simulink model "CurrentWithoutSim"  (R2022b)
settings: Solver=VariableStepAuto  StartTime=0.0  StopTime=20  RelTol=1e-3
PreLoadFcn:
  | openManipulatorParameters;
PostLoadFcn:
  | % Insert Communication Stuff Here
StartFcn:
  | myDxl.doEnableTorque(11);
  | myDxl.doEnableTorque(12);
  | myDxl.doEnableTorque(13);
  | myDxl.doEnableTorque(14);
  | myDxl.doEnableTorque(15);
StopFcn:
  | myDxl.doDisableTorque(11);
  | myDxl.doDisableTorque(12);
  | myDxl.doDisableTorque(13);
  | myDxl.doDisableTorque(14);
  | myDxl.doDisableTorque(15);
undefined symbols (not defined in the file): group_num_read, group_num_write, TsCtrl
libraries: slDxl_lib x12, dxlSimLibrary x2, OpenManipulatorLib x1
CloseFcn:
  | myDxl.delete()
settings Model: Creator=scastro  LastModifiedBy=Boog
settings SolverCC: AlgebraicLoopSolver=TrustRegion  DecoupledContinuousIntegration=on  MinimalZcImpactIntegration=on
settings DataIOCC: ReturnWorkspaceOutputs=off
settings DebuggingCC: ParameterOverflowMsg=none  UnconnectedInputMsg=warning  UnconnectedOutputMsg=warning  UnconnectedLineMsg=warning  SFMachineParentedDataDiag=warning  ArithmeticOperatorsInVariantConditions=warning
settings ModelReferenceCC: EnableRefExpFcnMdlSchedulingChecks=on
settings SFSimCC: SimUseLocalCustomCode=off  CustomCodeUndefinedFunction=UseInterfaceOnly
settings RTWCC: RTWUseLocalCustomCode=off
settings ExplorerConfigSet: InternalSimMechanicsExplorerSettings="<ExplorerConfiguration><canonicalview>default</canonicalview><AnimationSetting><BasePlaybackSpeed>1.0</BasePlaybackSpeed><PlaybackSpeedFactor>1.0</PlaybackSpeedFactor></AnimationSetting><TilePanel><TileInfo><Tiles Columns=\"1\" Count=\"1\" Rows=\"1\"><Column Weight=\"1\"/><Row Weight=\"1\"/><Tile Height=\"1\" Width=\"1\" X=\"0\" Y=\"0\"/></Tiles></TileInfo><SceneInfo><SceneViewer><BGColor><R>0.60000002384185791</R><G>0.60000002384185791</G><B>0.60000002384185791</B></BGColor><Camera><DoPerspective>off</DoPerspective><Position><X>0.428752942017998073</X><Y>-0.712150369953937545</Y><Z>0.628314823463847372</Z></Position><Center><X>0.0455703138120887447</X><Y>0.0802507835591396851</Y><Z>0.153687090021758288</Z></Center><Up><X>-0.128866037345358619</X><Y>0.462960972240881619</Y><Z>0.876961049648547597</Z></Up><ViewLimDist>1</ViewLimDist><YLim>0.579070269035580121</YLim><XLim>0.64437894599448009</XLim></Camera></SceneViewer></SceneInfo></TilePanel><MechEditorPanel><Cameras/><GfxPanelCameraMap/><VideoCreator><PlaybackSpeedRatio>1.0</PlaybackSpeedRatio><FrameRate>30</FrameRate><VideoFormat>Motion JPEG AVI</VideoFormat><FrameSize>auto</FrameSize></VideoCreator></MechEditorPanel></ExplorerConfiguration>"

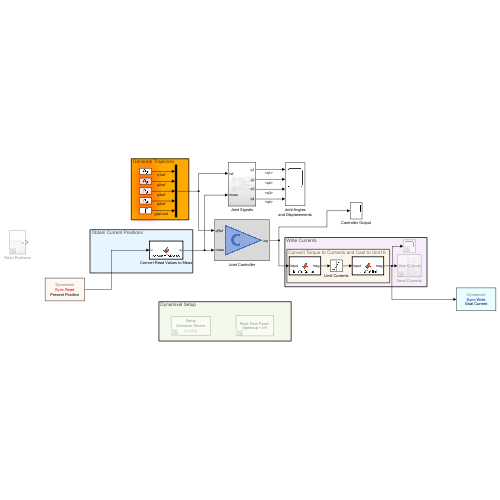
[thumbnail: Simulink's stored preview of the top-level diagram]
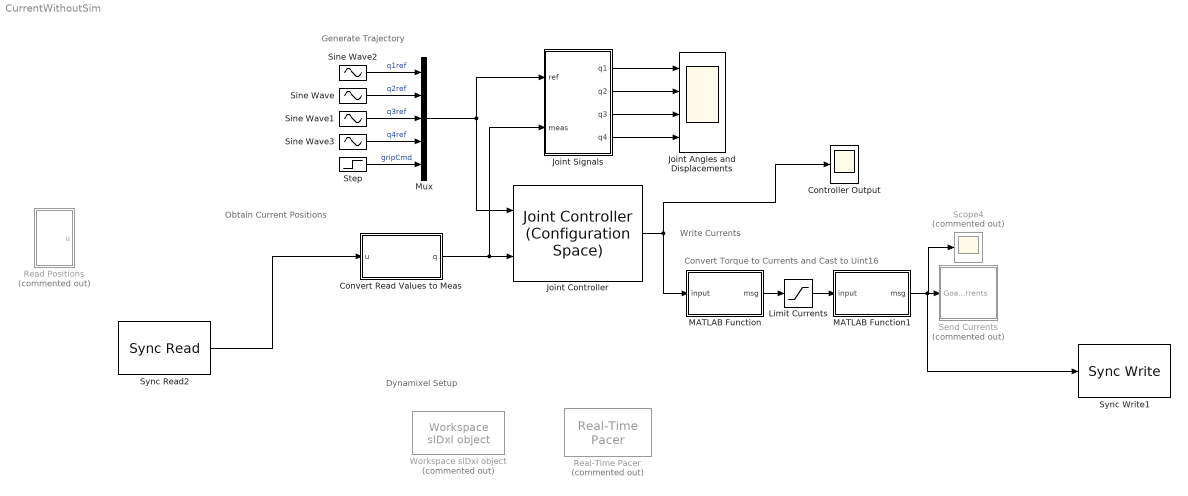
== system CurrentWithoutSim ==
  note: Dynamixel Setup
  note: Obtain Current Positions
  note: Write Currents
  note: Convert Torque to Currents and Cast to Uint16
  note: Generate Trajectory
  Controller Output : Scope
  Convert Read Values to Meas : MATLAB Function  TreatAsAtomicUnit=on
  Joint Angles and Displacements : Scope  NumInputPorts=4
  Joint Controller : OpenManipulatorLib/Joint Controller (Configuration Space)  SystemSampleTime=-1  VariantControl=ctrlType==1  VariantActivationTime=update diagram  Latency=0  AutoFrameSizeCalculation=off
      link override Saturate Inputs/Saturate  Joint Torques: UpperLimit=ctrlUpperLimit  LowerLimit=ctrlLowerLimit
  Joint Signals : Subsystem
  Limit Currents : Saturate  UpperLimit=50  LowerLimit=-50  OutDataTypeStr=int16
  MATLAB Function : MATLAB Function  TreatAsAtomicUnit=on
  MATLAB Function1 : MATLAB Function  TreatAsAtomicUnit=on
  Mux : Mux  Inputs=5
  Read Positions : Subsystem  Commented=on
  Real-Time Pacer : slDxl_lib/Real-Time Pacer  Commented=on  simTimePerRealTime=inf
  Scope4 : Scope  Commented=on
  Send Currents : Subsystem  Commented=on
  Sine Wave : Sin  Amplitude=pi/4  Frequency=0.2  SampleTime=TsCtrl
  Sine Wave1 : Sin  Amplitude=pi/5  Frequency=0.4  SampleTime=TsCtrl
  Sine Wave2 : Sin  Amplitude=2*pi/3  Frequency=.4  SampleTime=TsCtrl
  Sine Wave3 : Sin  Amplitude=pi/3  Frequency=0.25  SampleTime=TsCtrl
  Step : Step  Time=5  SampleTime=TsCtrl
  Sync Read2 : dxlSimLibrary/Sync Read  lib_name=lib_name  group_num=group_num_read(1)  ids=motor_IDs  models=motor_models  select=Present Position  Ts=0.005
  Sync Write1 : dxlSimLibrary/Sync Write  lib_name=lib_name  group_num=group_num_write(1)  ids=motor_IDs  models=motor_models  select=Goal Current  Ts=0.005
  Workspace slDxl object : slDxl_lib/Workspace slDxl object  Commented=on  slDxlVarName=Existing Object Handle #1  workspaceVarName=myDxl
  wires:
  Sine Wave/1 -> Mux/2  "q2ref"
  Sine Wave1/1 -> Mux/3  "q3ref"
  Sine Wave2/1 -> Mux/1  "q1ref"
  Mux/1 -> Joint Controller/1, Joint Signals/1(ref)
  Joint Signals/1(q1) -> Joint Angles and Displacements/1
  Joint Signals/2(q2) -> Joint Angles and Displacements/2
  Joint Signals/3(q3) -> Joint Angles and Displacements/3
  Joint Signals/4(q4) -> Joint Angles and Displacements/4
  Sine Wave3/1 -> Mux/4  "q4ref"
  Step/1 -> Mux/5  "gripCmd"
  Joint Controller/1 -> MATLAB Function/1(input), Controller Output/1
  Convert Read Values to Meas/1(q) -> Joint Controller/2, Joint Signals/2(meas)
  Limit Currents/1 -> MATLAB Function1/1(input)
  MATLAB Function1/1(msg) -> Sync Write1/1, Scope4/1, Send Currents/1(Goal Currents)
  MATLAB Function/1(msg) -> Limit Currents/1
  Sync Read2/1 -> Convert Read Values to Meas/1(u)

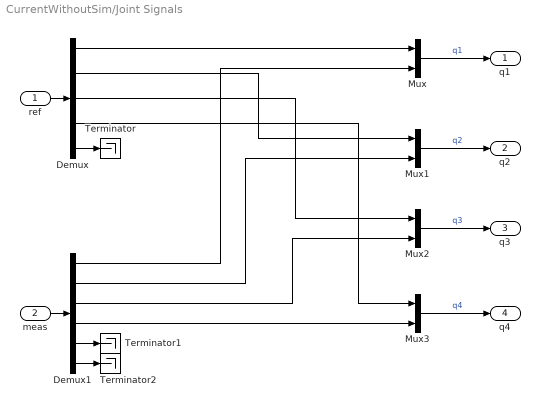
== system CurrentWithoutSim/Joint Signals ==
  ref : Inport
  meas : Inport  Port=2
  Demux : Demux  Outputs=5
  Demux1 : Demux  Outputs=6
  Mux{,1..3} (4 alike) : Mux  Inputs=2
  Terminator : Terminator
  Terminator1 : Terminator
  Terminator2 : Terminator
  q1 : Outport  VectorParamsAs1DForOutWhenUnconnected=off
  q2 : Outport  Port=2  VectorParamsAs1DForOutWhenUnconnected=off
  q3 : Outport  Port=3  VectorParamsAs1DForOutWhenUnconnected=off
  q4 : Outport  Port=4  VectorParamsAs1DForOutWhenUnconnected=off
  wires:
  Mux2/1 -> q3/1  "q3"
  ref/1 -> Demux/1
  Mux3/1 -> q4/1  "q4"
  Mux/1 -> q1/1  "q1"
  meas/1 -> Demux1/1
  Demux/1 -> Mux/1
  Demux1/1 -> Mux/2
  Mux1/1 -> q2/1  "q2"
  Demux/2 -> Mux1/1
  Demux1/2 -> Mux1/2
  Demux/3 -> Mux2/1
  Demux1/3 -> Mux2/2
  Demux1/4 -> Mux3/2
  Demux/4 -> Mux3/1
  Demux/5 -> Terminator/1
  Demux1/5 -> Terminator1/1
  Demux1/6 -> Terminator2/1

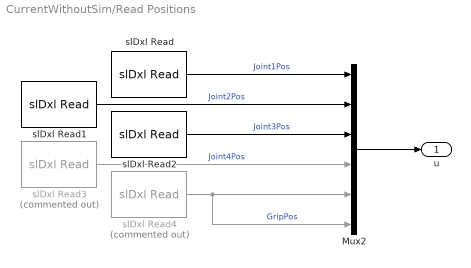
== system CurrentWithoutSim/Read Positions ==
  Mux2 : Mux  Inputs=6
  slDxl Read : slDxl_lib/slDxl Read  slDxlObject=Existing Object Handle #1  DXL_ID=11  DXL_ADDR=132  DXL_READ_SIZE=4  sampleT=-1
  slDxl Read1 : slDxl_lib/slDxl Read  slDxlObject=Existing Object Handle #1  DXL_ID=12  DXL_ADDR=132  DXL_READ_SIZE=4  sampleT=-1
  slDxl Read2 : slDxl_lib/slDxl Read  slDxlObject=Existing Object Handle #1  DXL_ID=13  DXL_ADDR=132  DXL_READ_SIZE=4  sampleT=-1
  slDxl Read3 : slDxl_lib/slDxl Read  Commented=on  slDxlObject=Existing Object Handle #1  DXL_ID=14  DXL_ADDR=132  DXL_READ_SIZE=4  sampleT=-1
  slDxl Read4 : slDxl_lib/slDxl Read  Commented=on  slDxlObject=Existing Object Handle #1  DXL_ID=15  DXL_ADDR=132  DXL_READ_SIZE=4  sampleT=Ts
  u : Outport
  wires:
  slDxl Read1/1 -> Mux2/2  "Joint2Pos"
  slDxl Read3/1 -> Mux2/4  "Joint4Pos"
  slDxl Read4/1 -> Mux2/6, Mux2/5  "GripPos"
  slDxl Read/1 -> Mux2/1  "Joint1Pos"
  slDxl Read2/1 -> Mux2/3  "Joint3Pos"
  Mux2/1 -> u/1

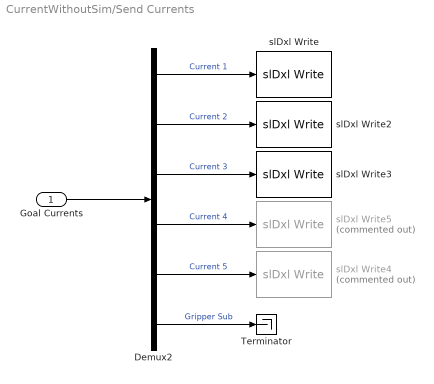
== system CurrentWithoutSim/Send Currents ==
  Goal Currents : Inport
  Demux2 : Demux  Outputs=6
  Terminator : Terminator
  slDxl Write : slDxl_lib/slDxl Write  slDxlObject=Existing Object Handle #1  DXL_ID=11  DXL_ADDR=102  DXL_WRITE_SIZE=2  sampleT=-1
  slDxl Write2 : slDxl_lib/slDxl Write  slDxlObject=Existing Object Handle #1  DXL_ID=12  DXL_ADDR=102  DXL_WRITE_SIZE=2  sampleT=-1
  slDxl Write3 : slDxl_lib/slDxl Write  slDxlObject=Existing Object Handle #1  DXL_ID=13  DXL_ADDR=102  DXL_WRITE_SIZE=2  sampleT=-1
  slDxl Write4 : slDxl_lib/slDxl Write  Commented=on  slDxlObject=Existing Object Handle #1  DXL_ID=15  DXL_ADDR=102  DXL_WRITE_SIZE=2  sampleT=Ts
  slDxl Write5 : slDxl_lib/slDxl Write  Commented=on  slDxlObject=Existing Object Handle #1  DXL_ID=14  DXL_ADDR=102  DXL_WRITE_SIZE=2  sampleT=-1
  wires:
  Demux2/6 -> Terminator/1  "Gripper Sub"
  Demux2/3 -> slDxl Write3/1  "Current 3"
  Demux2/2 -> slDxl Write2/1  "Current 2"
  Goal Currents/1 -> Demux2/1
  Demux2/4 -> slDxl Write5/1  "Current 4"
  Demux2/1 -> slDxl Write/1  "Current 1"
  Demux2/5 -> slDxl Write4/1  "Current 5"

== matlab function CurrentWithoutSim/MATLAB Function ==
  data: input input; msg output
function msg = tauToCurrent(input)
    current_A = 0.5714 .* input;
    msg = current_A .* 1000 ./ 2.69;

== matlab function CurrentWithoutSim/Convert Read Values to Meas ==
  data: u input; q output
function q = convertToMeas(u)
% 3.14 / 2048
q = (0.001534355386369.*u) - 3.14;

== matlab function CurrentWithoutSim/MATLAB Function1 ==
  data: input input; msg output
function msg = castToUint(input)
    msg = zeros(size(input));
    for i = 1:length(input)
        msg(i) = typecast(int16(input(i)), "uint16");
    end
end
